simulink model "ship_location_measurements_model_final"  (R2023b)
settings: Solver=VariableStepAuto  StartTime=0.0  StopTime=25  RelTol=1e-3
InitFcn:
  | dt=1;
settings Model: Creator=Noy Kirshner  LastModifiedBy=Noy Kirshner
settings SolverCC: AlgebraicLoopSolver=TrustRegion
settings RTWCC: DLArmComputeVersion=19.05

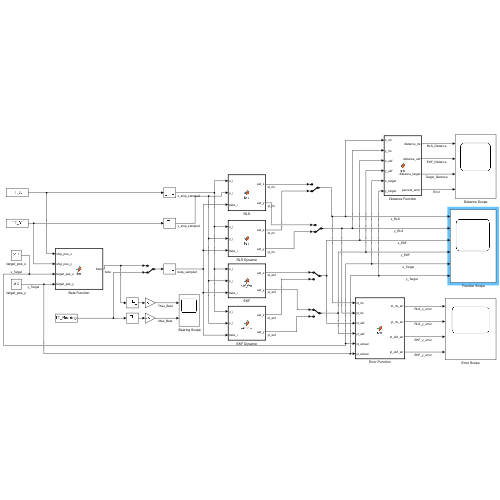
[thumbnail: Simulink's stored preview of the top-level diagram]
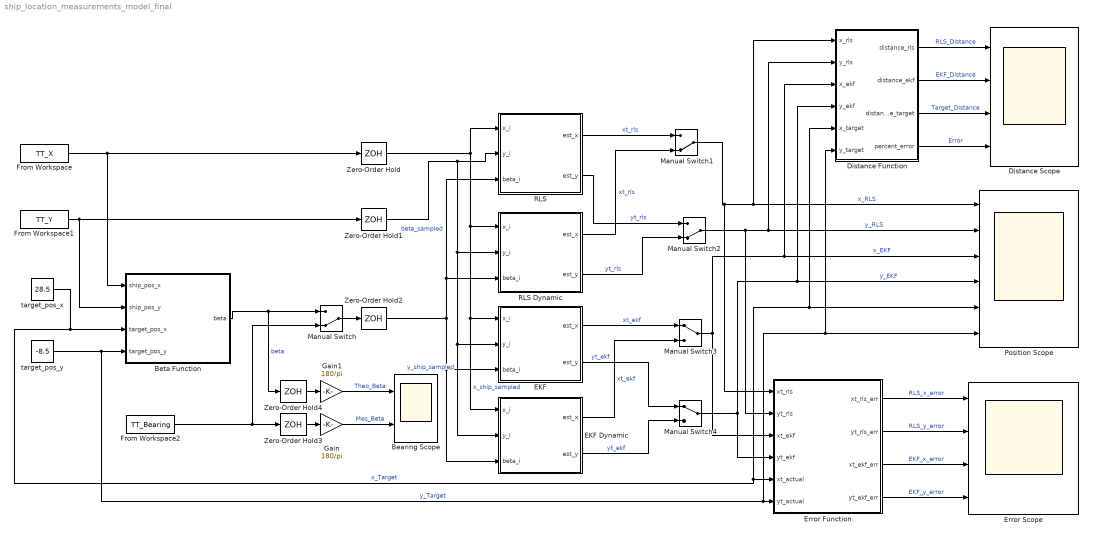
== system ship_location_measurements_model_final ==
  " Bearing Scope" : Scope  NumInputPorts=2
  " Position Scope" : Scope  NumInputPorts=6
  Beta Function : MATLAB Function  TreatAsAtomicUnit=on
  Distance Function : MATLAB Function  TreatAsAtomicUnit=on
  Distance Scope : Scope  NumInputPorts=4
  EKF : MATLAB Function  TreatAsAtomicUnit=on
  EKF Dynamic : MATLAB Function  TreatAsAtomicUnit=on
  Error Function : MATLAB Function  TreatAsAtomicUnit=on
  Error Scope : Scope  NumInputPorts=4
  From Workspace : FromWorkspace  VariableName=TT_X
  From Workspace1 : FromWorkspace  VariableName=TT_Y
  From Workspace2 : FromWorkspace  VariableName=TT_Bearing
  Gain : Gain  Gain=180/pi
  Gain1 : Gain  Gain=180/pi
  Manual Switch : ManualSwitch  CurrentSetting=0
  Manual Switch1 : ManualSwitch  CurrentSetting=0
  Manual Switch2 : ManualSwitch  CurrentSetting=0
  Manual Switch3 : ManualSwitch
  Manual Switch4 : ManualSwitch
  RLS : MATLAB Function  TreatAsAtomicUnit=on
  RLS Dynamic : MATLAB Function  TreatAsAtomicUnit=on
  Zero-Order Hold{,1..4} (5 alike) : ZeroOrderHold  SampleTime=dt
  target_pos_x : Constant  Value=28.5
  target_pos_y : Constant  Value=-8.5
  wires:
  target_pos_y/1 -> " Position Scope"/6, Distance Function/6(y_target), Error Function/6(yt_actual), Beta Function/4(target_pos_y)  "y_Target"
  target_pos_x/1 -> Distance Function/5(x_target), " Position Scope"/5, Error Function/5(xt_actual), Beta Function/3(target_pos_x)  "x_Target"
  Error Function/2(yt_rls_err) -> Error Scope/2  "RLS_y_error"
  Error Function/1(xt_rls_err) -> Error Scope/1  "RLS_x_error"
  Error Function/3(xt_ekf_err) -> Error Scope/3  "EKF_x_error"
  Error Function/4(yt_ekf_err) -> Error Scope/4  "EKF_y_error"
  Zero-Order Hold/1 -> EKF Dynamic/1(x_i), EKF/1(x_i), RLS Dynamic/1(x_i), RLS/1(x_i)  "x_ship_sampled"
  Zero-Order Hold1/1 -> EKF Dynamic/2(y_i), EKF/2(y_i), RLS Dynamic/2(y_i), RLS/2(y_i)  "y_ship_sampled"
  Zero-Order Hold2/1 -> EKF Dynamic/3(beta_i), EKF/3(beta_i), RLS Dynamic/3(beta_i), RLS/3(beta_i)  "beta_sampled"
  Manual Switch/1 -> Zero-Order Hold2/1
  From Workspace2/1 -> Manual Switch/2, Zero-Order Hold3/1
  Beta Function/1(beta) -> Zero-Order Hold4/1, Manual Switch/1  "beta"
  From Workspace1/1 -> Beta Function/2(ship_pos_y), Zero-Order Hold1/1
  From Workspace/1 -> Beta Function/1(ship_pos_x), Zero-Order Hold/1
  RLS/1(est_x) -> Manual Switch1/1  "xt_rls"
  RLS/2(est_y) -> Manual Switch2/1  "yt_rls"
  RLS Dynamic/1(est_x) -> Manual Switch1/2  "xt_rls"
  RLS Dynamic/2(est_y) -> Manual Switch2/2  "yt_rls"
  EKF/1(est_x) -> Manual Switch3/1  "xt_ekf"
  EKF Dynamic/1(est_x) -> Manual Switch3/2  "xt_ekf"
  EKF Dynamic/2(est_y) -> Manual Switch4/2  "yt_ekf"
  EKF/2(est_y) -> Manual Switch4/1  "yt_ekf"
  Manual Switch1/1 -> Error Function/1(xt_rls), Distance Function/1(x_rls), " Position Scope"/1  "x_RLS"
  Manual Switch2/1 -> Error Function/2(yt_rls), Distance Function/2(y_rls), " Position Scope"/2  "y_RLS"
  Manual Switch3/1 -> Distance Function/3(x_ekf), " Position Scope"/3, Error Function/3(xt_ekf)  "x_EKF"
  Manual Switch4/1 -> Error Function/4(yt_ekf), Distance Function/4(y_ekf), " Position Scope"/4  "y_EKF"
  Zero-Order Hold3/1 -> Gain/1
  Gain/1 -> " Bearing Scope"/2  "Mes_Beta"
  Gain1/1 -> " Bearing Scope"/1  "Theo_Beta"
  Zero-Order Hold4/1 -> Gain1/1
  Distance Function/1(distance_rls) -> Distance Scope/1  "RLS_Distance"
  Distance Function/2(distance_ekf) -> Distance Scope/2  "EKF_Distance"
  Distance Function/3(distance_target) -> Distance Scope/3  "Target_Distance"
  Distance Function/4(percent_error) -> Distance Scope/4  "Error"

== matlab function ship_location_measurements_model_final/Beta Function ==
  data: ship_pos_x input; beta output; ship_pos_y input; target_pos_x input; target_pos_y input
function beta = fcn(ship_pos_x,ship_pos_y,target_pos_x,target_pos_y)

dx = target_pos_x - ship_pos_x;
dy = target_pos_y - ship_pos_y;

beta = atan2(dy,dx);

== matlab function ship_location_measurements_model_final/RLS Dynamic ==
  data: x_i input; est_x output; y_i input; beta_i input; est_y output
function [est_x, est_y] = fcn(x_i, y_i, beta_i)

persistent P X_i lambda lambda_o

if isempty(P)
    P = eye(2);  % Covariance matrix initialization
    lambda_o = 0.8;
    lambda = 0.5;
end

if isempty(X_i)
    X_i = zeros(2, 1);  % X vector initialization as a zero vector
end


phi_i = [-sin(beta_i); cos(beta_i)]; % Update phi vector
z_i = y_i * cos(beta_i) - x_i * sin(beta_i); % z_i 
e = z_i - phi_i' * X_i; % update error vector
X_i = X_i + P * phi_i / (lambda + phi_i' * P * phi_i) * e; % Update X vector

g_k = P * phi_i / (lambda + phi_i' * P * phi_i); % Weight vector
P = (1 / lambda)* (P - g_k * phi_i' * P); % Covariance matrix update with forgetting factor
lambda = lambda_o*lambda + (1 -lambda_o);

% Update estimated position
est_x = X_i(1);
est_y = X_i(2);

end

== matlab function ship_location_measurements_model_final/RLS ==
  data: x_i input; est_x output; y_i input; beta_i input; est_y output
function [est_x, est_y] = fcn(x_i, y_i, beta_i)

persistent P X_i
gamma=0.55;
if isempty(P)
    P = eye(2);  % Covariance matrix initialization
end

if isempty(X_i)
    X_i = zeros(2, 1);  % X vector initialization as a zero vector
end

phi_i = [-sin(beta_i); cos(beta_i)]; % Update phi vector
z_i = y_i * cos(beta_i) - x_i * sin(beta_i); % z_i 
e = z_i - phi_i' * X_i; % update error vector
X_i = X_i + P * phi_i / (gamma + phi_i' * P * phi_i) * e; % Update X vector

g_k = P * phi_i / (1 + phi_i' * P * phi_i); % Weight vector
P = P - g_k * phi_i' * P; % Covariance matrix update

% Update estimated position
est_x = X_i(1);
est_y = X_i(2);

end

== matlab function ship_location_measurements_model_final/Error Function ==
  data: xt_rls input; xt_rls_err output; yt_rls input; xt_ekf input; yt_ekf input; xt_actual input; yt_actual input; yt_rls_err output; xt_ekf_err output; yt_ekf_err output
function [xt_rls_err,yt_rls_err,xt_ekf_err,yt_ekf_err] = fcn(xt_rls,yt_rls,xt_ekf,yt_ekf,xt_actual,yt_actual)

% RLS error values:
xt_rls_err = ((xt_rls - xt_actual)/xt_actual)*100;
yt_rls_err = ((yt_rls - yt_actual)/yt_actual)*100;

% EKF error values:
xt_ekf_err = ((xt_ekf - xt_actual)/xt_actual)*100;
yt_ekf_err = ((yt_ekf - yt_actual)/yt_actual)*100;

== matlab function ship_location_measurements_model_final/EKF ==
  data: x_i input; est_x output; y_i input; beta_i input; est_y output
function [est_x, est_y] = ekf_fcn(x_i, y_i, beta_i)

persistent X_i P Q R

if isempty(P)
    P = 1000000*eye(6); % Covariance matrix initialization (6x6)
    Q = 100*diag([0.01, 0.01, 1, 0.01, 1, 0.01]); % Process noise covariance initialization (6x6)
    R = 0.01*diag([1, 1, 100000]); % Measurement noise covariance initialization (3x3)
end

if isempty(X_i)
    X_i = zeros(6, 1); % State vector initialization (6x1)
end

dt = 1; % Sample time variable
F = [1 0 0 0 0 0 ; 0 1 0 0 0 0 ; 0 0 1 dt 0 0 ; 0 0 0 1 0 0 ; 0 0 0 0 1 dt ; 0 0 0 0 0 1]; % Process Jacobian (6x6)
H = [0 0 1 0 0 0 ; 0 0 0 0 1 0 ; sin(beta_i) -cos(beta_i) -sin(beta_i) 0 cos(beta_i) 0]; % Measurement Jacobian (3x6)

% Prediction Step
X_i = F*X_i; % Process Model
meas = [x_i ; y_i ; 0]; % Measurements
y_hat = H*X_i; % Measurement Model
P = F*P*F' + Q; % Covariance matrix

% Update Step
resid = meas - y_hat; % Measurement residual
K = P*H'/(H*P*H' + R); % Kalman gain
X_i = X_i + K*resid; % State vector update
P = (eye(6) - K*H)*P; % Covariance matrix update

% Output estimated position
est_x = X_i(1); % x_t estimation
est_y = X_i(2); % y_t estimation

end

== matlab function ship_location_measurements_model_final/EKF Dynamic ==
  data: x_i input; est_x output; y_i input; beta_i input; est_y output
function [est_x, est_y] = ekf_fcn(x_i, y_i, beta_i)

persistent X_i P Q R

if isempty(P)
    P = 1000000000*eye(8); % Covariance matrix initialization (8x8)
    Q = 10000*diag([1, 0.01, 1, 0.01, 1, 0.01, 1, 0.01]); % Process noise covariance initialization (8x8)
    R = diag([10, 10, 40000000]); % Measurement noise covariance initialization (3x3)
end
 
if isempty(X_i)
    X_i = zeros(8, 1); % State vector initialization (8x1)
end

dt = 0.001; % Sample time variable
F = [1 dt 0 0 0 0 0 0 ; 0 1 0 0 0 0 0 0 ; 0 0 1 dt 0 0 0 0 ; 0 0 0 1 0 0 0 0 ; 0 0 0 0 1 dt 0 0 ; 0 0 0 0 0 1 0 0 ; 0 0 0 0 0 0 1 dt ; 0 0 0 0 0 0 0 1]; % Process Jacobian (8x8)
H = [0 0 0 0 1 0 0 0 ; 0 0 0 0 0 0 1 0 ; sin(beta_i) 0 -cos(beta_i) 0 -sin(beta_i) 0 cos(beta_i) 0]; % Measurement Jacobian (3x8)

% Prediction Step
X_i = F*X_i; % Process Model
meas = [x_i ; y_i ; 0]; % Measurements
y_hat = H*X_i; % Measurement Model
P = F*P*F' + Q; % Covariance matrix

% Update Step
resid = meas - y_hat; % Measurement residual
K = P*H'/(H*P*H' + R); % Kalman gain
X_i = X_i + K*resid; % State vector update
P = (eye(8) - K*H)*P; % Covariance matrix update

% Output estimated position
est_x = X_i(1); % x_t estimation
est_y = X_i(3); % y_t estimation

end

== matlab function ship_location_measurements_model_final/Distance Function ==
  data: x_rls input; distance_rls output; y_rls input; x_ekf input; y_ekf input; distance_ekf output; x_target input; y_target input; distance_target output; percent_error output
function [distance_rls,distance_ekf,distance_target,percent_error]= fcn(x_rls,y_rls,x_ekf,y_ekf,x_target,y_target)

distance_rls = sqrt(x_rls^2 + y_rls^2);
distance_ekf = sqrt(x_ekf^2 + y_ekf^2);
distance_target = sqrt(x_target^2 + y_target^2);
percent_error = 0.9*distance_target;
